simulink model "AllPurposeModel_TyreRelaxation_CreateBusFormats"  (R2014b)
settings: Solver=ode45  StartTime=0.0  StopTime=10.0  MaxStep=0.01  RelTol=1e-3
InitFcn:
  | %clear;
  | %load('vectors_busformats.mat')
StartFcn:
  | %clear;
  | %BJ_test_init;
settings Model: Creator=bengtja  LastModifiedBy=Daniel
settings DebuggingCC: UnderspecifiedInitializationDetection=Classic  MergeDetectMultiDrivingBlocksExec=none

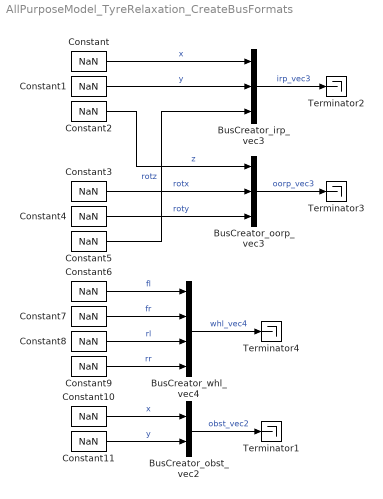
== system AllPurposeModel_TyreRelaxation_CreateBusFormats ==
  BusCreator_irp_vec3 : BusCreator  Inputs=3
  BusCreator_obst_vec2 : BusCreator  Inputs=2
  BusCreator_oorp_vec3 : BusCreator  Inputs=3
  BusCreator_whl_vec4 : BusCreator
  Constant{,1..11} (12 alike) : Constant  Value=NaN
  Terminator{1..4} (4 alike) : Terminator
  wires:
  Constant1/1 -> BusCreator_irp_vec3/2  "y"
  BusCreator_irp_vec3/1 -> Terminator2/1  "irp_vec3"
  Constant/1 -> BusCreator_irp_vec3/1  "x"
  BusCreator_oorp_vec3/1 -> Terminator3/1  "oorp_vec3"
  Constant4/1 -> BusCreator_oorp_vec3/3  "roty"
  Constant3/1 -> BusCreator_oorp_vec3/2  "rotx"
  Constant5/1 -> BusCreator_irp_vec3/3  "rotz"
  Constant2/1 -> BusCreator_oorp_vec3/1  "z"
  BusCreator_whl_vec4/1 -> Terminator4/1  "whl_vec4"
  Constant6/1 -> BusCreator_whl_vec4/1  "fl"
  Constant7/1 -> BusCreator_whl_vec4/2  "fr"
  Constant8/1 -> BusCreator_whl_vec4/3  "rl"
  Constant9/1 -> BusCreator_whl_vec4/4  "rr"
  BusCreator_obst_vec2/1 -> Terminator1/1  "obst_vec2"
  Constant10/1 -> BusCreator_obst_vec2/1  "x"
  Constant11/1 -> BusCreator_obst_vec2/2  "y"
